simulink model "tpec2022_dab_nn_openl"  (R2017b)
settings: Solver=FixedStepAuto  StartTime=0.0  StopTime=0.5  FixedStep=1e-6  MaxStep=1e-4  RelTol=1e-3
undefined symbols (not defined in the file or in its folder): d1, d2, phase
libraries: powerlib x20, powerlib_meascontrol x10
settings Model: Creator=mluser  LastModifiedBy=akarbozo
settings DataIOCC: ReturnWorkspaceOutputs=on
settings DebuggingCC: SFMachineParentedDataDiag=error
settings SFSimCC: SimUseLocalCustomCode=on
settings RTWCC: RTWUseLocalCustomCode=on

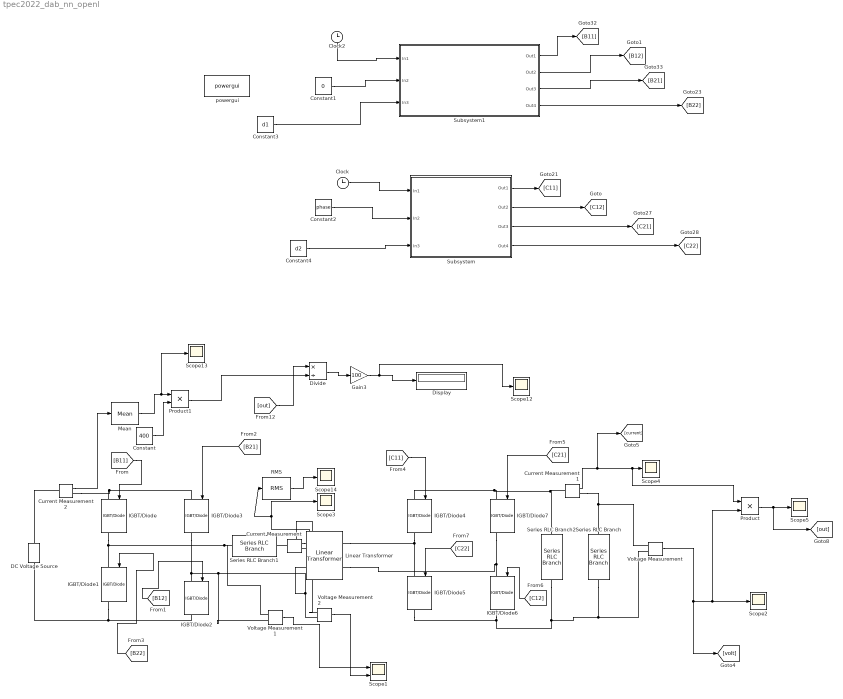
== system tpec2022_dab_nn_openl ==
  Clock : Clock
  Clock2 : Clock
  Constant : Constant  Value=400
  Constant1 : Constant  Value=0
  Constant2 : Constant  Value=phase
  Constant3 : Constant  Value=d1
  Constant4 : Constant  Value=d2
  Current Measurement : powerlib/Measurements/Current Measurement  PhasorSimulation=off  OutputType=Complex  PSBequivalent=0
  Current Measurement1 : powerlib/Measurements/Current Measurement  PhasorSimulation=off  OutputType=Complex  PSBequivalent=0
  Current Measurement2 : powerlib/Measurements/Current Measurement  PhasorSimulation=off  OutputType=Complex  PSBequivalent=0
  DC Voltage Source : powerlib/Electrical Sources/DC Voltage Source  Amplitude=400  Measurements=None
  Display : Display
  Divide : Product  Inputs=*/
  Gain3 : Gain  Gain=100
  IGBT/Diode{,1..7} (8 alike) : powerlib/Power Electronics/IGBT//Diode  Ron=1e-4  Rs=1e5  Cs=inf  Measurements=on
  Linear Transformer : powerlib/Elements/Linear Transformer  UNITS=SI  NominalPower=[300e3 50000 ]  winding1=[10000 0 0]  winding2=[10000 0 0]  ThreeWindings=off  winding3=[3.15e+05 793.8 0.10107]  RmLm=[2e+12 3.9789e+08]  Measurements=None  DataType=on
  Mean : powerlib_meascontrol/Measurements/Mean  Freq=50000  Vinit=0  Ts=0
  Product : Product
  Product1 : Product
  RMS : powerlib_meascontrol/Measurements/RMS  TrueRMS=on  Freq=50000  RMSInit=0  Ts=0
  Scope1 : Scope  NumInputPorts=2
  Scope{2..5,12..14} (7 alike) : Scope
  Series RLC Branch : powerlib/Elements/Series RLC Branch  LConnTagsString=__new0  RConnTagsString=__new0  BranchType=R  Resistance=400*400/100000  Inductance=1e-3  SetiL0=off  InitialCurrent=0  Capacitance=1e-6  Setx0=off  InitialVoltage=0  Measurements=None
  Series RLC Branch1 : powerlib/Elements/Series RLC Branch  LConnTagsString=__new0  RConnTagsString=__new0  BranchType=RL  Resistance=0.5  Inductance=2.42649e-6  SetiL0=off  InitialCurrent=0  Capacitance=1e-6  Setx0=off  InitialVoltage=0  Measurements=None
  Series RLC Branch2 : powerlib/Elements/Series RLC Branch  LConnTagsString=__new0  RConnTagsString=__new0  BranchType=RC  Resistance=1e-6  Inductance=1e-3  SetiL0=off  InitialCurrent=0  Capacitance=10e-3  Setx0=off  InitialVoltage=0  Measurements=None
  Subsystem : Subsystem
  Subsystem1 : Subsystem
  Voltage Measurement : powerlib/Measurements/Voltage Measurement  PhasorSimulation=off  OutputType=Complex  PSBequivalent=0
  Voltage Measurement1 : powerlib/Measurements/Voltage Measurement  PhasorSimulation=off  OutputType=Complex  PSBequivalent=0
  Voltage Measurement2 : powerlib/Measurements/Voltage Measurement  PhasorSimulation=off  OutputType=Complex  PSBequivalent=0
  powergui : powerlib/powergui  Priority=1  SimulationMode=Discrete  SampleTime=1e-6  frequency=60  Iterations=50  frequencyindice=0  Pbase=100e6  ErrMax=1e-4  UnitsV=kV  UnitsW=MW  buscounter=0  FunctionMessages=off  echomessages=off  EnableUseOfTLC=off  CurrentSourceSwitches=off  DisableSnubberDevices=off  DisableRonSwitches=off  DisableVfSwitches=off  DisplayEquations=off  SolverType=Tustin/Backward Euler (TBE)  Interpol=off  ExternalGateDelay=off  methode=off  Ts=100  x0status=blocks  SPID=off  SwTol=0  HookPort=off  RestoreLinks=warning  ResistiveCurrentMeasurement=off  Frange=[0:2:500]  Ylog=off  Xlog=on  ShowGrid=off  save=off  variable=ZData  structure=0  ZoomFFT=off  StartTime=0.0  cycles=1  DisplayStyle=1  fundamental=60  FreqAxis=off  MaxFrequency=1000  frequencyindicesteady=1  RmsSteady=1  display=off
  wires:
  RMS/1 -> Scope14/1
  Current Measurement2/1 -> Mean/1
  [C12] -> IGBT/Diode6/1
  Constant/1 -> Product1/2
  [C11] -> IGBT/Diode4/1
  [B11] -> IGBT/Diode/1
  Mean/1 -> Scope13/1, Product1/1
  [C21] -> IGBT/Diode7/1
  [out] -> Divide/1
  [B21] -> IGBT/Diode3/1
  [B22] -> IGBT/Diode1/1
  [C22] -> IGBT/Diode5/1
  Gain3/1 -> Scope12/1, Display/1
  Product1/1 -> Divide/2
  Current Measurement1/1 -> [current], Product/1, Scope4/1
  Voltage Measurement/1 -> Product/2, Scope2/1, [volt]
  Divide/1 -> Gain3/1
  Voltage Measurement1/1 -> Scope1/1
  Product/1 -> [out], Scope5/1
  Voltage Measurement2/1 -> Scope1/2
  Current Measurement/1 -> RMS/1, Scope3/1
  [B12] -> IGBT/Diode2/1
  Subsystem/1(Out1) -> [C11]
  Constant1/1 -> Subsystem1/2(In2)
  Clock2/1 -> Subsystem1/1(In1)
  Constant2/1 -> Subsystem/2(In2)
  Subsystem1/3(Out3) -> [B21]
  Clock/1 -> Subsystem/1(In1)
  Subsystem/4(Out4) -> [C22]
  Subsystem1/2(Out2) -> [B12]
  Subsystem/3(Out3) -> [C21]
  Subsystem1/1(Out1) -> [B11]
  Subsystem/2(Out2) -> [C12]
  Subsystem1/4(Out4) -> [B22]
  Constant4/1 -> Subsystem/3(In3)
  Constant3/1 -> Subsystem1/3(In3)
  connections:
  Voltage Measurement1/LConn1 -- IGBT/Diode1/LConn1 -- IGBT/Diode/RConn1 -- Series RLC Branch1/LConn1
  Linear Transformer/LConn1 -- Current Measurement/RConn1 -- Voltage Measurement2/LConn1
  Voltage Measurement1/LConn2 -- Voltage Measurement2/LConn2 -- Linear Transformer/LConn2 -- IGBT/Diode3/RConn1 -- IGBT/Diode2/LConn1
  Current Measurement1/RConn1 -- Voltage Measurement/LConn1 -- Series RLC Branch/LConn1
  Linear Transformer/RConn1 -- IGBT/Diode5/LConn1 -- IGBT/Diode4/RConn1
  IGBT/Diode5/RConn1 -- IGBT/Diode6/RConn1 -- Series RLC Branch2/RConn1 -- Series RLC Branch/RConn1 -- Voltage Measurement/LConn2
  Current Measurement2/RConn1 -- IGBT/Diode3/LConn1 -- IGBT/Diode/LConn1
  Current Measurement1/LConn1 -- IGBT/Diode7/LConn1 -- IGBT/Diode4/LConn1 -- Series RLC Branch2/LConn1
  Linear Transformer/RConn2 -- IGBT/Diode7/RConn1 -- IGBT/Diode6/LConn1
  DC Voltage Source/LConn1 -- IGBT/Diode2/RConn1 -- IGBT/Diode1/RConn1
  Current Measurement2/LConn1 -- DC Voltage Source/RConn1
  Current Measurement/LConn1 -- Series RLC Branch1/RConn1

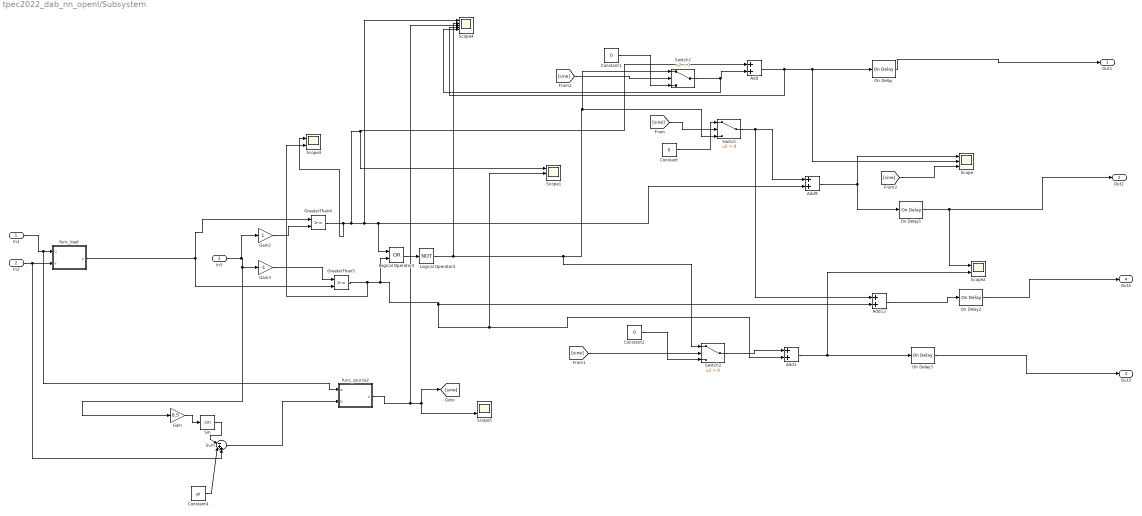
== system tpec2022_dab_nn_openl/Subsystem ==
  In1 : Inport
  In2 : Inport  Port=2
  In3 : Inport  Port=3
  Add{,1,9,12} (4 alike) : Sum
  Constant : Constant  Value=0
  Constant1 : Constant  Value=0
  Constant2 : Constant  Value=0
  Constant4 : Constant  Value=pi
  Gain : Gain  Gain=0.5
  Gain2 : Gain
  Gain3 : Gain  Gain=-1
  GreaterThan4 : RelationalOperator  OutDataTypeStr=boolean  RndMeth=Simplest
  GreaterThan5 : RelationalOperator  OutDataTypeStr=boolean  RndMeth=Simplest
  Logical Operator3 : Logic  Operator=OR  AllPortsSameDT=off  OutDataTypeStr=boolean
  Logical Operator4 : Logic  Operator=NOT  AllPortsSameDT=off  OutDataTypeStr=boolean
  On Delay{,1..3} (4 alike) : powerlib_meascontrol/Logic/On Delay  DelayType=On delay  delay=0  ic=0  Ts=0
      settings: SourceProductName=Simscape Power Systems
  Scope : Scope  NumInputPorts=3
  Scope1 : Scope  NumInputPorts=3
  Scope2 : Scope  NumInputPorts=2
  Scope3 : Scope  NumInputPorts=2
  Scope4 : Scope  NumInputPorts=5
  Scope5 : Scope  NumInputPorts=2
  Sin : Trigonometry
  Sum : Sum  Inputs=|-++
  Switch : Switch  Criteria=u2 > Threshold
  Switch1 : Switch  Criteria=u2 > Threshold
  Switch2 : Switch  Criteria=u2 > Threshold
  func_load : MATLAB Function  TreatAsAtomicUnit=on
  func_source2 : MATLAB Function  TreatAsAtomicUnit=on
  Out1 : Outport
  Out2 : Outport  Port=2
  Out3 : Outport  Port=3
  Out4 : Outport  Port=4
  wires:
  [sine] -> Scope/3
  Gain2/1 -> GreaterThan4/2
  Add/1 -> Scope4/4, On Delay/1, Scope/2
  Add1/1 -> Scope2/2, On Delay3/1
  Add9/1 -> On Delay1/1, Scope/1
  On Delay/1 -> Out1/1
  Add12/1 -> On Delay2/1
  Switch/1 -> Add12/1, Add9/1
  Logical Operator3/1 -> Logical Operator4/1
  Switch2/1 -> Add1/1
  [sine] -> Switch/2
  [sine] -> Switch1/2
  GreaterThan5/1 -> Scope3/2, Scope1/2, Add1/2, Add12/2, Logical Operator3/2
  Logical Operator4/1 -> Scope4/2, Switch2/1, Switch/3, Switch1/1
  Gain3/1 -> GreaterThan5/1
  func_load/1(y) -> GreaterThan5/2, GreaterThan4/1
  [sine] -> Switch2/2
  On Delay3/1 -> Out3/1
  On Delay2/1 -> Out4/1
  On Delay1/1 -> Out2/1, Scope2/1
  GreaterThan4/1 -> Scope3/1, Add/1, Scope1/1, Scope4/1, Add9/2, Logical Operator3/1
  In1/1 -> func_source2/1(a), func_load/1(u)
  Switch1/1 -> Scope4/5, Add/2
  func_source2/1(z) -> Scope4/3, [sine], Scope5/2
  Sum/1 -> func_source2/2(b)
  In2/1 -> Sum/3, func_load/2(v)
  Constant1/1 -> Switch1/3
  Constant2/1 -> Switch2/3
  Constant/1 -> Switch/1
  Constant4/1 -> Sum/2
  Gain/1 -> Sin/1
  In3/1 -> Gain2/1, Gain/1, Gain3/1
  Sin/1 -> Sum/1

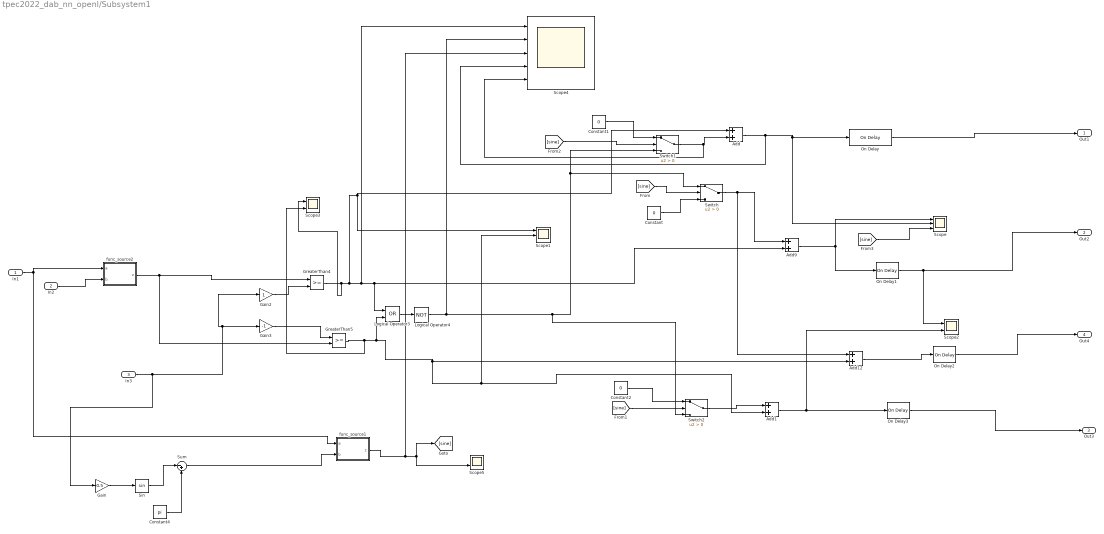
== system tpec2022_dab_nn_openl/Subsystem1 ==
  In1 : Inport
  In2 : Inport  Port=2
  In3 : Inport  Port=3
  Add{,1,9,12} (4 alike) : Sum
  Constant : Constant  Value=0
  Constant1 : Constant  Value=0
  Constant2 : Constant  Value=0
  Constant4 : Constant  Value=pi
  Gain : Gain  Gain=0.5
  Gain2 : Gain
  Gain3 : Gain  Gain=-1
  GreaterThan4 : RelationalOperator  OutDataTypeStr=boolean  RndMeth=Simplest
  GreaterThan5 : RelationalOperator  OutDataTypeStr=boolean  RndMeth=Simplest
  Logical Operator3 : Logic  Operator=OR  AllPortsSameDT=off  OutDataTypeStr=boolean
  Logical Operator4 : Logic  Operator=NOT  AllPortsSameDT=off  OutDataTypeStr=boolean
  On Delay{,1..3} (4 alike) : powerlib_meascontrol/Logic/On Delay  DelayType=On delay  delay=0  ic=0  Ts=0
      settings: SourceProductName=Simscape Power Systems
  Scope : Scope  NumInputPorts=3
  Scope1 : Scope  NumInputPorts=3
  Scope2 : Scope  NumInputPorts=2
  Scope3 : Scope  NumInputPorts=2
  Scope4 : Scope  NumInputPorts=5
  Scope5 : Scope  NumInputPorts=2
  Sin : Trigonometry
  Sum : Sum  Inputs=|-+
  Switch : Switch  Criteria=u2 > Threshold
  Switch1 : Switch  Criteria=u2 > Threshold
  Switch2 : Switch  Criteria=u2 > Threshold
  func_source1 : MATLAB Function  TreatAsAtomicUnit=on
  func_source2 : MATLAB Function  TreatAsAtomicUnit=on
  Out1 : Outport
  Out2 : Outport  Port=2
  Out3 : Outport  Port=3
  Out4 : Outport  Port=4
  wires:
  [sine] -> Scope/3
  Gain2/1 -> GreaterThan4/2
  Add/1 -> Scope4/4, Scope/2, On Delay/1
  Add1/1 -> Scope2/2, On Delay3/1
  Add9/1 -> On Delay1/1, Scope/1
  On Delay/1 -> Out1/1
  Add12/1 -> On Delay2/1
  Switch/1 -> Add12/1, Add9/1
  Logical Operator3/1 -> Logical Operator4/1
  Switch2/1 -> Add1/1
  [sine] -> Switch/2
  [sine] -> Switch1/2
  GreaterThan5/1 -> Scope3/2, Scope1/2, Add1/2, Add12/2, Logical Operator3/2
  Logical Operator4/1 -> Scope4/2, Switch2/3, Switch/1, Switch1/3
  Gain3/1 -> GreaterThan5/1
  In3/1 -> Gain/1, Gain3/1, Gain2/1
  [sine] -> Switch2/2
  On Delay3/1 -> Out3/1
  On Delay2/1 -> Out4/1
  On Delay1/1 -> Out2/1, Scope2/1
  GreaterThan4/1 -> Scope3/1, Add/1, Scope1/1, Scope4/1, Add9/2, Logical Operator3/1
  In1/1 -> func_source1/1(a), func_source2/1(a)
  Switch1/1 -> Scope4/5, Add/2
  func_source1/1(z) -> Scope4/3, [sine], Scope5/2
  Sum/1 -> func_source1/2(b)
  func_source2/1(z) -> GreaterThan5/2, GreaterThan4/1
  In2/1 -> func_source2/2(b)
  Constant1/1 -> Switch1/1
  Constant/1 -> Switch/3
  Constant2/1 -> Switch2/1
  Gain/1 -> Sin/1
  Constant4/1 -> Sum/2
  Sin/1 -> Sum/1

== matlab function tpec2022_dab_nn_openl/Subsystem/func_load ==
  data: u input; y output; v input
function y = fcn(u,v)
%#codegen

y = sin(2*pi*f*u - v );
end

== matlab function tpec2022_dab_nn_openl/Subsystem1/func_source2 ==
  data: a input; z output; b input
function z = fcn(a,b)
%#codegen

z = sin(2*pi*f*a - b);
end

== matlab function tpec2022_dab_nn_openl/Subsystem/func_source2 ==
  data: a input; z output; b input
function z = fcn(a,b)
%#codegen

z = sin(2*pi*f*a - b);
end

== matlab function tpec2022_dab_nn_openl/Subsystem1/func_source1 ==
  data: a input; z output; b input
function z = fcn(a,b)
%#codegen

z = sin(2*pi*f*a - b);
end
